simulink model "sum"  (Simulink 7.3)
settings: Solver=ode45  StartTime=0.0  StopTime=10.0  RelTol=1e-3
libraries: simulink x1
settings Model: Creator=Achyut  LastModifiedBy=Achyut

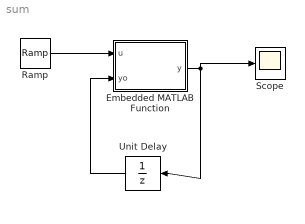
== system sum ==
  Embedded MATLAB Function : Stateflow chart
  Ramp : simulink/Sources/Ramp  SystemSampleTime=-1  slope=1  start=0  X0=0
  Scope : Scope
  Unit Delay : UnitDelay  SampleTime=-1
  wires:
  Embedded MATLAB Function/1(y) -> Unit Delay/1, Scope/1
  Unit Delay/1 -> Embedded MATLAB Function/2(yo)
  Ramp/1 -> Embedded MATLAB Function/1(u)

== matlab function Embedded MATLAB Function ==
  data: u input double; y output double; yo input double
function y = fcn(u,yo)
%#eml

y = u+yo;
